simulink model "Car15WithArduinoPin"  (R2024a)
settings: Solver=FixedStepAuto  StartTime=0.0  StopTime=inf  RelTol=1e-3  EnableMultiTasking=on
model workspace (MAT data in the model file):
  indicator = -1
libraries: arduinolib x15
settings Model: ExtModeTrigDuration=2  Creator=thipp  LastModifiedBy=thipp
settings SolverCC: AutoInsertRateTranBlk=on
settings OptimizationCC: EnhancedBackFolding=on  PassReuseOutputArgsAs=Individual arguments  ZeroExternalMemoryAtStartup=off  ZeroInternalMemoryAtStartup=off  MaxStackSize=64  OptimizeBlockOrder=speed  DifferentSizesBufferReuse=on  OptimizationCustomize=off  EfficientTunableParamExpr=on
settings DebuggingCC: ParameterTunabilityLossMsg=error
settings HardwareCC: ProdBitPerInt=16  ProdBitPerPointer=16  ProdBitPerSizeT=16  ProdBitPerPtrDiffT=16  ProdLargestAtomicFloat=None  ProdWordSize=8  ProdHWDeviceType=Atmel->AVR  UseEmbeddedCoderFeatures=off  UseSimulinkCoderFeatures=off
settings SFSimCC: MATLABDynamicMemAlloc=off
settings RTWCC: Description=Embedded Coder  SystemTargetFile=ert.tlc  HardwareBoard=Arduino Mega 2560  TemplateMakefile=ert_default_tmf  Toolchain=Arduino AVR  BuildConfiguration=Faster Runs
settings CodeAppCC: ForceParamTrailComments=on  IgnoreCustomStorageClasses=off  OperatorAnnotations=on  SimulinkDataObjDesc=on  SFDataObjDesc=on  InsertBlockDesc=on
settings ERTTargetCC: SupportContinuousTime=on  SupportNonInlinedSFcns=on  SupportVariableSizeSignals=on  ExtModeTransport=3  ExtModeStaticAlloc=on  ExtModeAutomaticAllocSize=off  ExtModeStaticAllocSize=2048  ExtModeMexFile=ext_xcp  ExtModeIntrfLevel=Level2 - Open

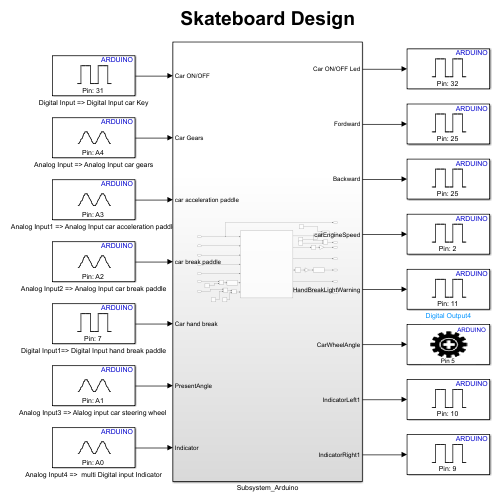
[thumbnail: Simulink's stored preview of the top-level diagram]
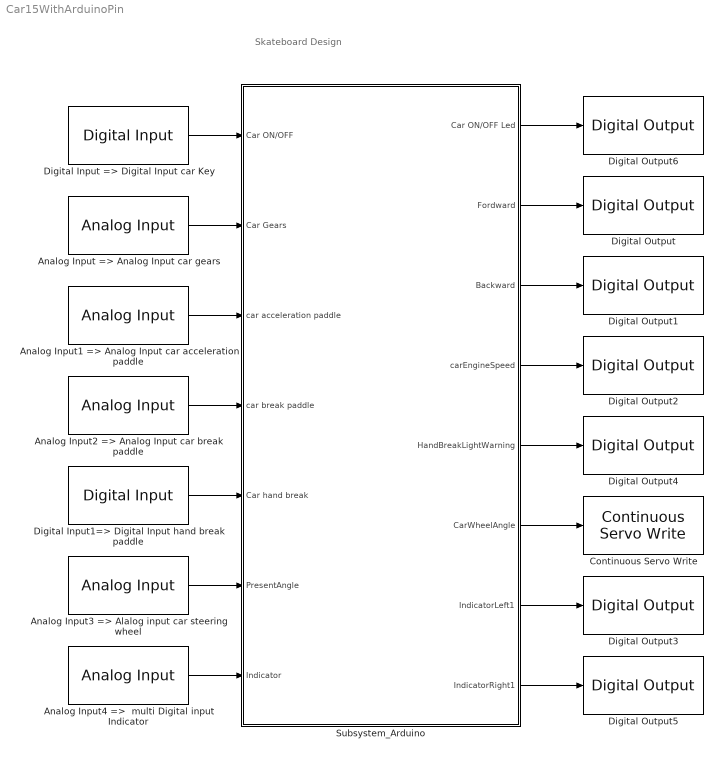
== system Car15WithArduinoPin ==
  note: Skateboard Design
  Analog Input => Analog Input car gears : arduinolib/Analog Input  pinNumber=4  ReadResultsOnly=off  ConversionTriggerSource=Software  ExternalTriggerType=uint32( 0 )  OutputDataType=uint16  EnableConversionCompleteNotify=off  EnableOuputStatus=off  SampleTime=-1  blockPlatform=arduino
  Analog Input1 => Analog Input car acceleration paddle : arduinolib/Analog Input  pinNumber=3  ReadResultsOnly=off  ConversionTriggerSource=Software  ExternalTriggerType=uint32( 0 )  OutputDataType=uint16  EnableConversionCompleteNotify=off  EnableOuputStatus=off  SampleTime=-1  blockPlatform=arduino
  Analog Input2 => Analog Input car break paddle : arduinolib/Analog Input  pinNumber=2  ReadResultsOnly=off  ConversionTriggerSource=Software  ExternalTriggerType=uint32( 0 )  OutputDataType=uint16  EnableConversionCompleteNotify=off  EnableOuputStatus=off  SampleTime=-1  blockPlatform=arduino
  "Analog Input3 => Alalog input car steering wheel " : arduinolib/Analog Input  pinNumber=1  ReadResultsOnly=off  ConversionTriggerSource=Software  ExternalTriggerType=uint32( 0 )  OutputDataType=uint16  EnableConversionCompleteNotify=off  EnableOuputStatus=off  SampleTime=-1  blockPlatform=arduino
  Analog Input4 =>  multi Digital input Indicator : arduinolib/Analog Input  pinNumber=0  ReadResultsOnly=off  ConversionTriggerSource=Software  ExternalTriggerType=uint32( 0 )  OutputDataType=uint16  EnableConversionCompleteNotify=off  EnableOuputStatus=off  SampleTime=-1  blockPlatform=arduino
  Continuous Servo Write : arduinolib/Continuous Servo Write  pinNumber=5  ServoIndex=0  blockPlatform=ARDUINO
  Digital Input => Digital Input car Key : arduinolib/Digital Input  pinNumber=31  mode=Input Pullup  Direction=input  SampleTime=0.1  blockPlatform=arduino
  Digital Input1=> Digital Input hand break paddle : arduinolib/Digital Input  pinNumber=7  mode=Default  Direction=input  SampleTime=0.1  blockPlatform=arduino
  Digital Output : arduinolib/Digital Output  pinNumber=25  Direction=output  blockPlatform=arduino
  Digital Output1 : arduinolib/Digital Output  pinNumber=25  Direction=output  blockPlatform=arduino
  Digital Output2 : arduinolib/Digital Output  pinNumber=2  Direction=output  blockPlatform=arduino
  Digital Output3 : arduinolib/Digital Output  pinNumber=10  Direction=output  blockPlatform=arduino
  Digital Output4 : arduinolib/Digital Output  pinNumber=11  Direction=output  blockPlatform=arduino
  Digital Output5 : arduinolib/Digital Output  pinNumber=9  Direction=output  blockPlatform=arduino
  Digital Output6 : arduinolib/Digital Output  pinNumber=32  Direction=output  blockPlatform=arduino
  Subsystem_Arduino : Subsystem
  wires:
  Digital Input => Digital Input car Key/1 -> Subsystem_Arduino/1(Car ON/OFF)
  Analog Input => Analog Input car gears/1 -> Subsystem_Arduino/2(Car Gears)
  Analog Input1 => Analog Input car acceleration paddle/1 -> Subsystem_Arduino/3(car acceleration paddle)
  Analog Input2 => Analog Input car break paddle/1 -> Subsystem_Arduino/4(car break paddle)
  Digital Input1=> Digital Input hand break paddle/1 -> Subsystem_Arduino/5("Car hand break ")
  "Analog Input3 => Alalog input car steering wheel "/1 -> Subsystem_Arduino/6(PresentAngle)
  Analog Input4 =>  multi Digital input Indicator/1 -> Subsystem_Arduino/7(Indicator)
  Subsystem_Arduino/2(Fordward) -> Digital Output/1
  Subsystem_Arduino/3(Backward) -> Digital Output1/1
  Subsystem_Arduino/4(carEngineSpeed) -> Digital Output2/1
  Subsystem_Arduino/5(HandBreakLightWarning) -> Digital Output4/1
  Subsystem_Arduino/6(CarWheelAngle) -> Continuous Servo Write/1
  Subsystem_Arduino/7(IndicatorLeft1) -> Digital Output3/1
  Subsystem_Arduino/8(IndicatorRight1) -> Digital Output5/1
  Subsystem_Arduino/1(Car ON/OFF Led) -> Digital Output6/1

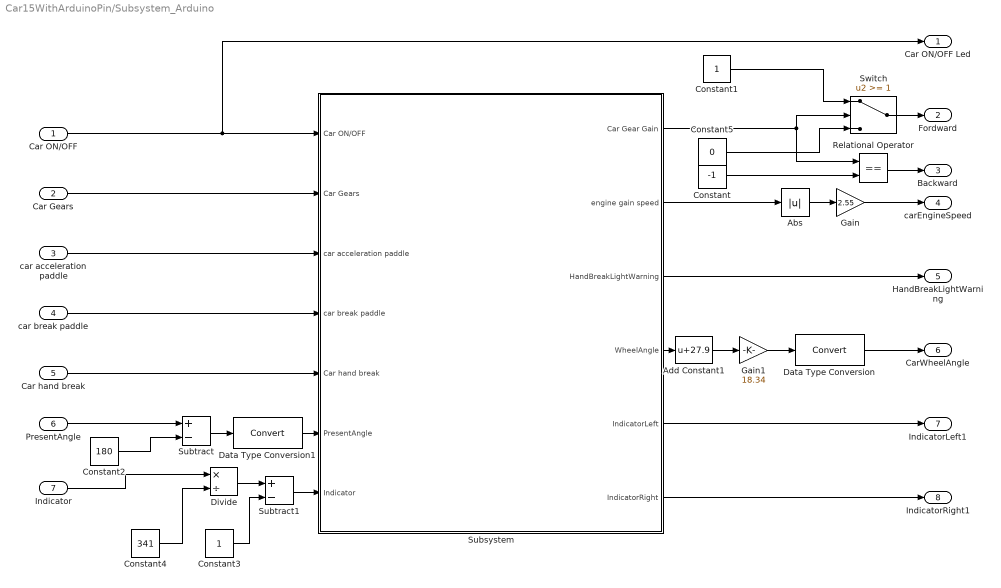
== system Car15WithArduinoPin/Subsystem_Arduino ==
  Car ON/OFF : Inport
  Car Gears : Inport  Port=2
  car acceleration paddle : Inport  Port=3
  car break paddle : Inport  Port=4
  "Car hand break " : Inport  Port=5
  PresentAngle : Inport  Port=6
  Indicator : Inport  Port=7
  Abs : Abs  SaturateOnIntegerOverflow=off
  Add Constant1 : Bias  Bias=27.9  SaturateOnIntegerOverflow=off
  Constant : Constant  Value=-1
  Constant1 : Constant
  Constant2 : Constant  Value=180
  Constant3 : Constant
  Constant4 : Constant  Value=341
  Constant5 : Constant  Value=0
  Data Type Conversion : DataTypeConversion  RndMeth=Ceiling  SaturateOnIntegerOverflow=off
  Data Type Conversion1 : DataTypeConversion  SaturateOnIntegerOverflow=off  RndMeth=Floor
  Divide : Product  Inputs=*/
  Gain : Gain  Gain=2.55
  Gain1 : Gain  Gain=18.34
  Relational Operator : RelationalOperator  Operator===  OutDataTypeStr=boolean  RndMeth=Simplest  InputSameDT=off
  Subsystem : Subsystem
  Subtract : Sum  Inputs=+-
  Subtract1 : Sum  Inputs=+-
  Switch : Switch  Threshold=1  SaturateOnIntegerOverflow=off  InputSameDT=off
  Car ON/OFF Led : Outport
  Fordward : Outport  Port=2
  Backward : Outport  Port=3
  carEngineSpeed : Outport  Port=4
  HandBreakLightWarning : Outport  Port=5
  CarWheelAngle : Outport  Port=6
  IndicatorLeft1 : Outport  Port=7
  IndicatorRight1 : Outport  Port=8
  wires:
  Divide/1 -> Subtract1/1
  Subsystem/3(HandBreakLightWarning) -> HandBreakLightWarning/1
  Subsystem/4(WheelAngle) -> Add Constant1/1
  Subsystem/2(engine gain speed) -> Abs/1
  Constant4/1 -> Divide/2
  Subsystem/6(IndicatorRight) -> IndicatorRight1/1
  Subsystem/5(IndicatorLeft) -> IndicatorLeft1/1
  Subtract/1 -> Data Type Conversion1/1
  Subtract1/1 -> Subsystem/7(Indicator)
  Add Constant1/1 -> Gain1/1
  Constant3/1 -> Subtract1/2
  Indicator/1 -> Divide/1
  Gain/1 -> carEngineSpeed/1
  PresentAngle/1 -> Subtract/1
  car break paddle/1 -> Subsystem/4(car break paddle)
  Gain1/1 -> Data Type Conversion/1
  Abs/1 -> Gain/1
  Data Type Conversion1/1 -> Subsystem/6(PresentAngle)
  car acceleration paddle/1 -> Subsystem/3(car acceleration paddle)
  Constant2/1 -> Subtract/2
  "Car hand break "/1 -> Subsystem/5("Car hand break ")
  Data Type Conversion/1 -> CarWheelAngle/1
  Car Gears/1 -> Subsystem/2(Car Gears)
  Subsystem/1(Car Gear Gain) -> Relational Operator/1, Switch/2
  Switch/1 -> Fordward/1
  Constant1/1 -> Switch/1
  Relational Operator/1 -> Backward/1
  Constant5/1 -> Switch/3
  Constant/1 -> Relational Operator/2
  Car ON/OFF/1 -> Car ON/OFF Led/1, Subsystem/1(Car ON/OFF)

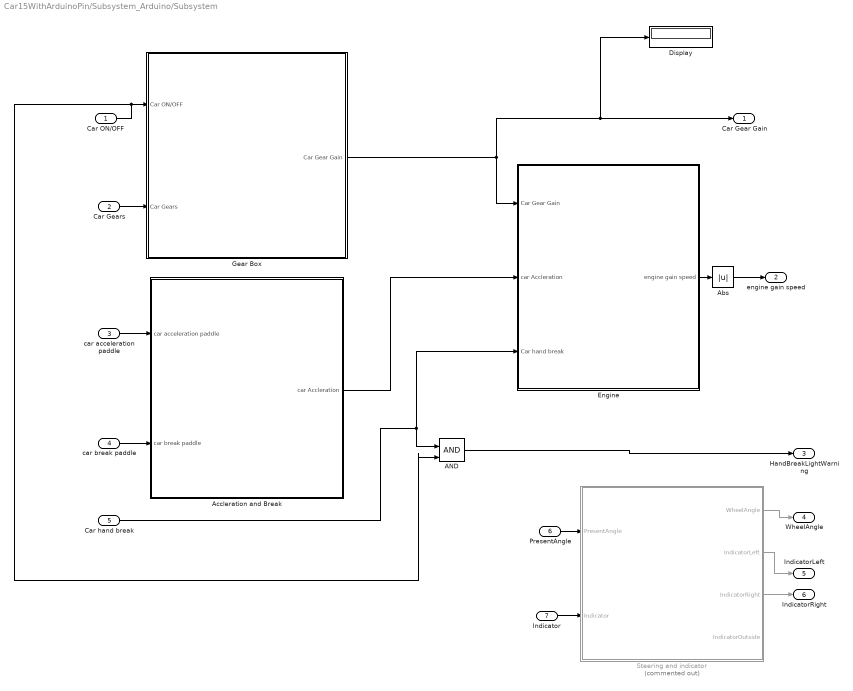
== system Car15WithArduinoPin/Subsystem_Arduino/Subsystem ==
  Car ON/OFF : Inport
  Car Gears : Inport  Port=2
  car acceleration paddle : Inport  Port=3
  car break paddle : Inport  Port=4
  "Car hand break " : Inport  Port=5
  PresentAngle : Inport  Port=6
  Indicator : Inport  Port=7
  AND : Logic  IconShape=distinctive  AllPortsSameDT=off  OutDataTypeStr=boolean
  Abs : Abs  SaturateOnIntegerOverflow=off
  Accleration and Break : Subsystem
  Display : Display
  Engine : Subsystem
  Gear Box : Subsystem
  "Steering and indicator " : Subsystem  Commented=on
  Car Gear Gain : Outport
  engine gain speed : Outport  Port=2
  HandBreakLightWarning : Outport  Port=3
  WheelAngle : Outport  Port=4
  IndicatorLeft : Outport  Port=5
  IndicatorRight : Outport  Port=6
  wires:
  Car ON/OFF/1 -> Gear Box/1(Car ON/OFF), AND/2
  Accleration and Break/1(car Accleration) -> Engine/2(car Accleration)
  "Steering and indicator "/3(IndicatorRight) -> IndicatorRight/1
  "Steering and indicator "/2(IndicatorLeft) -> IndicatorLeft/1
  car acceleration paddle/1 -> Accleration and Break/1(car acceleration paddle)
  Indicator/1 -> "Steering and indicator "/2(Indicator)
  "Car hand break "/1 -> Engine/3("Car hand break "), AND/1
  Engine/1(engine gain speed) -> Abs/1
  car break paddle/1 -> Accleration and Break/2(car break paddle)
  Car Gears/1 -> Gear Box/2(Car Gears)
  Abs/1 -> engine gain speed/1
  "Steering and indicator "/1(WheelAngle) -> WheelAngle/1
  AND/1 -> HandBreakLightWarning/1
  PresentAngle/1 -> "Steering and indicator "/1(PresentAngle)
  Gear Box/1(Car Gear Gain) -> Engine/1(Car Gear Gain), Display/1, Car Gear Gain/1

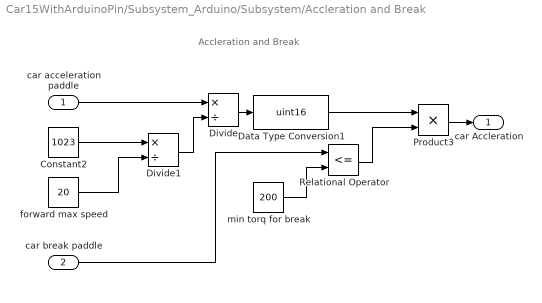
== system Car15WithArduinoPin/Subsystem_Arduino/Subsystem/Accleration and Break ==
  note: Accleration and Break
  car acceleration paddle : Inport
  car break paddle : Inport  Port=2
  Constant2 : Constant  Value=1023
  Data Type Conversion1 : DataTypeConversion  OutDataTypeStr=uint16  SaturateOnIntegerOverflow=off  RndMeth=Floor
  Divide : Product  Inputs=*/  RndMeth=Zero  SaturateOnIntegerOverflow=on
  Divide1 : Product  Inputs=*/  RndMeth=Zero  SaturateOnIntegerOverflow=on
  Product3 : Product
  Relational Operator : RelationalOperator  Operator=<=  OutDataTypeStr=boolean  RndMeth=Simplest  InputSameDT=off
  forward max speed : Constant  Value=20
  min torq for break : Constant  Value=200
  car Accleration : Outport
  wires:
  min torq for break/1 -> Relational Operator/2
  Divide/1 -> Data Type Conversion1/1
  forward max speed/1 -> Divide1/2
  car break paddle/1 -> Relational Operator/1
  Data Type Conversion1/1 -> Product3/1
  Constant2/1 -> Divide1/1
  Divide1/1 -> Divide/2
  Relational Operator/1 -> Product3/2
  car acceleration paddle/1 -> Divide/1
  Product3/1 -> car Accleration/1

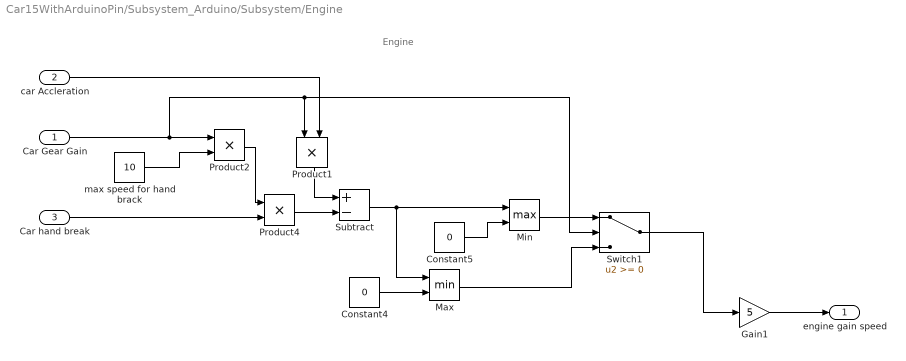
== system Car15WithArduinoPin/Subsystem_Arduino/Subsystem/Engine ==
  note: Engine
  Car Gear Gain : Inport
  car Accleration : Inport  Port=2
  "Car hand break " : Inport  Port=3
  Constant4 : Constant  Value=0
  Constant5 : Constant  Value=0
  Gain1 : Gain  Gain=5
  Max : MinMax  Inputs=2
  Min : MinMax  Function=max  Inputs=2
  Product1 : Product
  Product2 : Product
  Product4 : Product
  Subtract : Sum  Inputs=+-
  Switch1 : Switch  SaturateOnIntegerOverflow=off  InputSameDT=off
  max speed for hand brack : Constant  Value=10
  engine gain speed : Outport
  wires:
  Subtract/1 -> Min/1, Max/1
  Switch1/1 -> Gain1/1
  Product2/1 -> Product4/1
  Product1/1 -> Subtract/1
  Product4/1 -> Subtract/2
  Constant5/1 -> Min/2
  max speed for hand brack/1 -> Product2/2
  Car Gear Gain/1 -> Product1/1, Switch1/2, Product2/1
  Max/1 -> Switch1/3
  Min/1 -> Switch1/1
  Constant4/1 -> Max/2
  car Accleration/1 -> Product1/2
  "Car hand break "/1 -> Product4/2
  Gain1/1 -> engine gain speed/1

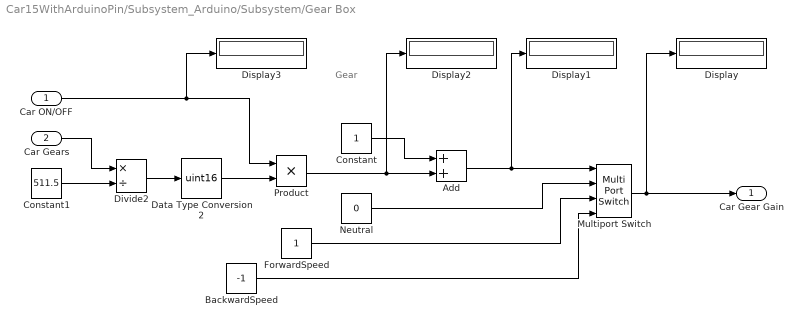
== system Car15WithArduinoPin/Subsystem_Arduino/Subsystem/Gear Box ==
  note: Gear
  Car ON/OFF : Inport
  Car Gears : Inport  Port=2
  Add : Sum
  BackwardSpeed : Constant  Value=-1
  Constant : Constant
  Constant1 : Constant  Value=511.5
  Data Type Conversion2 : DataTypeConversion  OutDataTypeStr=uint16  RndMeth=Nearest  SaturateOnIntegerOverflow=off
  Display{,1..3} (4 alike) : Display
  Divide2 : Product  Inputs=*/  RndMeth=Zero  SaturateOnIntegerOverflow=on
  ForwardSpeed : Constant
  Multiport Switch : MultiPortSwitch  SaturateOnIntegerOverflow=off  InputSameDT=off
  Neutral : Constant  Value=0
  Product : Product
  Car Gear Gain : Outport
  wires:
  Add/1 -> Display1/1, Multiport Switch/1
  Neutral/1 -> Multiport Switch/2
  Constant1/1 -> Divide2/2
  Product/1 -> Display2/1, Add/2
  BackwardSpeed/1 -> Multiport Switch/4
  Data Type Conversion2/1 -> Product/2
  ForwardSpeed/1 -> Multiport Switch/3
  Divide2/1 -> Data Type Conversion2/1
  Constant/1 -> Add/1
  Multiport Switch/1 -> Display/1, Car Gear Gain/1
  Car ON/OFF/1 -> Display3/1, Product/1
  Car Gears/1 -> Divide2/1

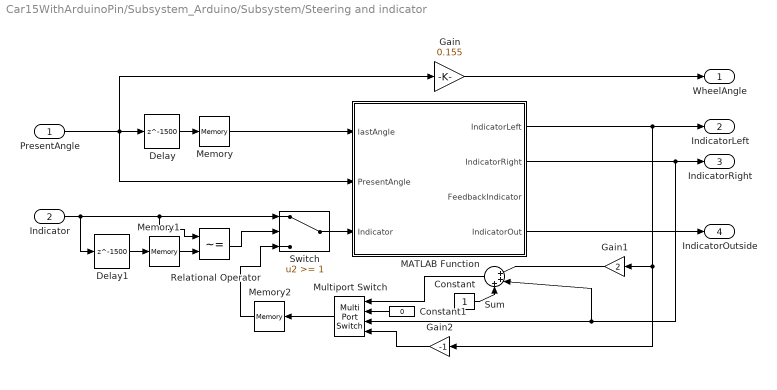
== system Car15WithArduinoPin/Subsystem_Arduino/Subsystem/Steering and indicator  ==
  PresentAngle : Inport
  Indicator : Inport  Port=2
  Constant : Constant
  Constant1 : Constant  Value=0
  Delay : Delay  DelayLength=1500
  Delay1 : Delay  DelayLength=1500
  Gain : Gain  Gain=0.155
  Gain1 : Gain  Gain=2
  Gain2 : Gain  Gain=-1
  MATLAB Function : MATLAB Function  TreatAsAtomicUnit=on
  Memory : Memory
  Memory1 : Memory
  Memory2 : Memory
  Multiport Switch : MultiPortSwitch  SaturateOnIntegerOverflow=off  InputSameDT=off
  Relational Operator : RelationalOperator  Operator=~=  OutDataTypeStr=boolean  RndMeth=Simplest  InputSameDT=off
  Sum : Sum  Inputs=|+++
  Switch : Switch  Threshold=1  SaturateOnIntegerOverflow=off  InputSameDT=off
  WheelAngle : Outport
  IndicatorLeft : Outport  Port=2
  IndicatorRight : Outport  Port=3
  IndicatorOutside : Outport  Port=4
  wires:
  PresentAngle/1 -> MATLAB Function/2(PresentAngle), Gain/1, Delay/1
  MATLAB Function/1(IndicatorLeft) -> Gain2/1, Gain1/1, IndicatorLeft/1
  Gain/1 -> WheelAngle/1
  Memory/1 -> MATLAB Function/1(lastAngle)
  Delay/1 -> Memory/1
  MATLAB Function/4(IndicatorOut) -> IndicatorOutside/1
  Indicator/1 -> Delay1/1, Relational Operator/1, Switch/1
  Relational Operator/1 -> Switch/2
  Switch/1 -> MATLAB Function/3(Indicator)
  Memory1/1 -> Relational Operator/2
  Delay1/1 -> Memory1/1
  Memory2/1 -> Switch/3
  Sum/1 -> Multiport Switch/1
  Constant/1 -> Sum/3
  Constant1/1 -> Multiport Switch/2
  MATLAB Function/2(IndicatorRight) -> Sum/2, Multiport Switch/3, IndicatorRight/1
  Gain1/1 -> Sum/1
  Gain2/1 -> Multiport Switch/4
  Multiport Switch/1 -> Memory2/1

== matlab function Car15WithArduinoPin/Subsystem_Arduino/Subsystem/Steering and indicator /MATLAB Function ==
  data: IndicatorLeft output; IndicatorRight output; FeedbackIndicator output; IndicatorOut output; lastAngle input; PresentAngle input; Indicator input
function [IndicatorLeft, IndicatorRight,FeedbackIndicator,IndicatorOut] = fcn(lastAngle, PresentAngle, Indicator)
    % Determine the turning direction
    turning = 0;
    if PresentAngle> lastAngle 
        turning = 1; % Turning right
    elseif PresentAngle< lastAngle 
        turning = -1; % Turning left
    end
    
    % Update the indicator position based on the turning direction
    IndicatorPosition = Indicator;
    if Indicator == 1 && turning == -1
        IndicatorPosition = 0; % Cancel right indicator when turning left
    elseif Indicator == -1 && turning == 1
        IndicatorPosition = 0; % Cancel left indicator when turning right
    end
    
    % Determine the state of left and right indicators
    LI = 0;
    RI = 0;
    FB = 0;
    if IndicatorPosition == -1
        LI = 1; % Left indicator is on
        FB=-1;
    end
    if IndicatorPosition == 1
        RI = 1; % Right indicator is on
        FB=1;
    end
    
    % Assign outputs
    IndicatorOut = IndicatorPosition;
    IndicatorLeft = LI;
    IndicatorRight = RI;
    FeedbackIndicator = FB;
end
